simulink model "reg_ze_sp_od_stanu"  (R2021a)
settings: Solver=VariableStepAuto  StartTime=0.0  StopTime=120  RelTol=1e-3
values from neighbouring files (symbols this model uses):
  k1 = k(1,1)    [liczenie_k.m]    (also in skrypt_k_i_l.m; zad4.m; zad_dod.m = K(1))
  k2 = k(1,2)    [liczenie_k.m]    (also in skrypt_k_i_l.m; zad4.m; zad_dod.m = K(2))
  k3 = k(1,3)    [liczenie_k.m]    (also in skrypt_k_i_l.m; zad4.m; zad_dod.m = K(3))
settings Model: Creator=ADMIN  LastModifiedBy=ADMIN

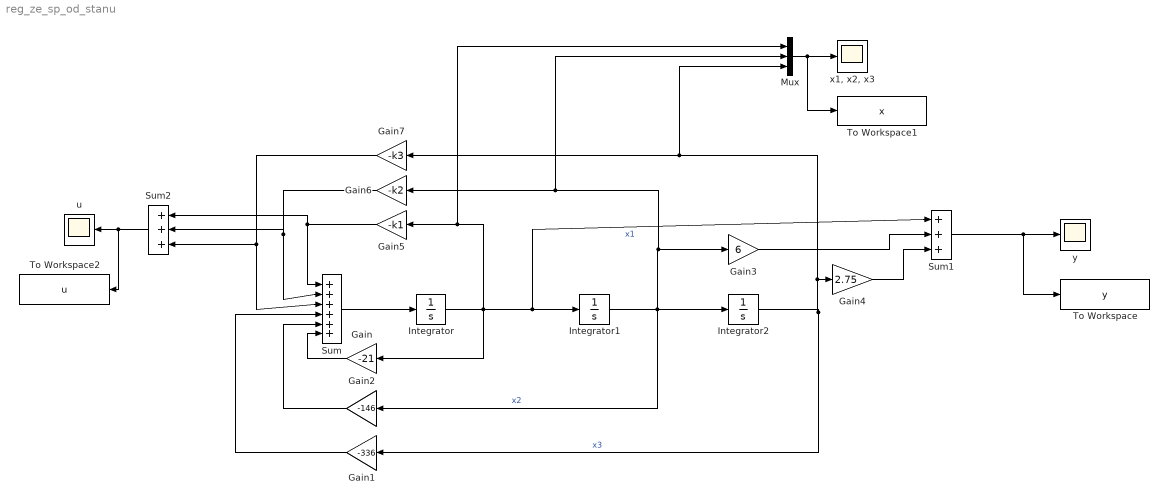
== system reg_ze_sp_od_stanu ==
  Gain : Gain  Gain=-21
  Gain1 : Gain  Gain=-336
  Gain2 : Gain  Gain=-146
  Gain3 : Gain  Gain=6
  Gain4 : Gain  Gain=2.75
  Gain5 : Gain  Gain=-k1
  Gain6 : Gain  Gain=-k2
  Gain7 : Gain  Gain=-k3
  Integrator : Integrator  InitialCondition=1
  Integrator1 : Integrator  InitialCondition=2
  Integrator2 : Integrator  InitialCondition=4
  Mux : Mux  Inputs=3
  Sum : Sum  Inputs=|++++++
  Sum1 : Sum  Inputs=|+++
  Sum2 : Sum  Inputs=|+++
  To Workspace : ToWorkspace  VariableName=y  SaveFormat=Structure With Time  SampleTime=-1
  To Workspace1 : ToWorkspace  VariableName=x  SaveFormat=Structure With Time  SampleTime=-1
  To Workspace2 : ToWorkspace  VariableName=u  SaveFormat=Structure With Time  SampleTime=-1
  u : Scope
  "x1, x2, x3" : Scope
  y : Scope
  wires:
  Sum1/1 -> To Workspace/1, y/1
  Gain3/1 -> Sum1/2
  Sum/1 -> Integrator/1
  Integrator1/1 -> Mux/2, Gain6/1, Gain3/1, Gain2/1, Integrator2/1  "x2"
  Integrator2/1 -> Mux/3, Gain7/1, Gain4/1, Gain1/1  "x3"
  Gain4/1 -> Sum1/3
  Gain2/1 -> Sum/5
  Gain1/1 -> Sum/4
  Integrator/1 -> Mux/1, Gain5/1, Sum1/1, Integrator1/1, Gain/1  "x1"
  Gain/1 -> Sum/6
  Gain5/1 -> Sum2/1, Sum/1
  Gain6/1 -> Sum2/2, Sum/2
  Gain7/1 -> Sum2/3, Sum/3
  Mux/1 -> To Workspace1/1, "x1, x2, x3"/1
  Sum2/1 -> To Workspace2/1, u/1
